simulink model "Ziegler_Nichols_PID"  (R2020b)
settings: Solver=VariableStepAuto  StartTime=0.0  StopTime=50  MaxStep=0.01  RelTol=1e-3
libraries: pid_lib x1
settings Model: Creator=amnessa  LastModifiedBy=amnessa

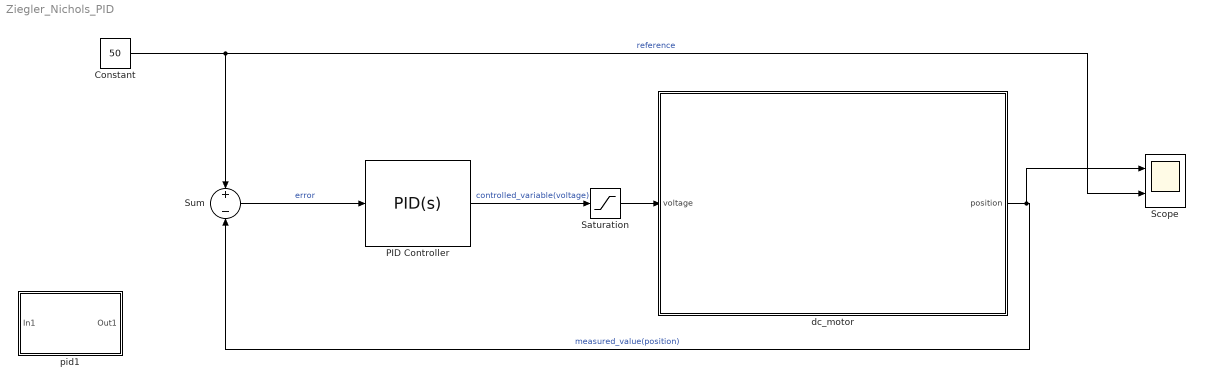
== system Ziegler_Nichols_PID ==
  Constant : Constant  Value=50
  PID Controller : pid_lib/PID Controller  Controller=PID  Form=Parallel  TimeDomain=Continuous-time  UseExternalTs=off  SampleTime=-1  IntegratorMethod=Forward Euler  FilterMethod=Forward Euler  ControllerParametersSource=internal  P=6.77668774596396  I=1.08320309237299  D=5.65172406078375  UseFilter=on  N=1208.48557960799  TunerSelectOption=Transfer Function Based (PID Tuner App)  InitialConditionSource=internal  InitialConditionForIntegrator=0  InitialConditionForFilter=0  DifferentiatorICPrevScaledInput=0  ExternalReset=none  TrackingMode=off  Kt=1  LimitOutput=off  SatLimitsSource=internal  UpperSaturationLimit=inf  LowerSaturationLimit=-inf  LinearizeAsGain=on  AntiWindupMode=none  Kb=1  POutMin=[]  POutMax=[]  IOutMin=[]  IOutMax=[]  DOutMin=[]  DOutMax=[]  NOutMin=[]  NOutMax=[]  SumOutMin=[]  SumOutMax=[]  SaturationOutMin=[]  SaturationOutMax=[]  PParamMin=[]  PParamMax=[]  IParamMin=[]  IParamMax=[]  DParamMin=[]  DParamMax=[]  NParamMin=[]  NParamMax=[]  KbParamMin=[]  KbParamMax=[]  KtParamMin=[]  KtParamMax=[]  KbOutMin=[]  KbOutMax=[]  KtOutMin=[]  KtOutMax=[]  IntegratorOutMin=[]  IntegratorOutMax=[]  FilterOutMin=[]  FilterOutMax=[]  SumI1OutMin=[]  SumI1OutMax=[]  SumI2OutMin=[]  SumI2OutMax=[]  SumI3OutMin=[]  SumI3OutMax=[]  SumI4OutMin=[]  SumI4OutMax=[]  SumDOutMin=[]  SumDOutMax=[]  DifferentiatorOutMin=[]  DifferentiatorOutMax=[]  FilterDiffOutCoefMin=[]  FilterDiffOutCoefMax=[]  ReciprocalOutMin=[]  ReciprocalOutMax=[]  SumDenOutMin=[]  SumDenOutMax=[]  SumNumOutMin=[]  SumNumOutMax=[]  DivideOutMin=[]  DivideOutMax=[]  UdiffTsProdOutMin=[]  UdiffTsProdOutMax=[]  NTsProdOutMin=[]  NTsProdOutMax=[]  UintegralTsProdOutMin=[]  UintegralTsProdOutMax=[]  UngainTsProdOutMin=[]  UngainTsProdOutMax=[]  IntegratorContinuousStateAttributes=''  IntegratorStateMustResolveToSignalObject=off  IntegratorRTWStateStorageClass=Auto  FilterContinuousStateAttributes=''  FilterStateMustResolveToSignalObject=off  FilterRTWStateStorageClass=Auto  ParallelPVariant=InternalParameters  IdealPVariant=Disabled  IVariant=InternalParameters  DVariant=InternalParameters  IntegratorVariant=Continuous  SatVariant=Disabled  AWVariant=Passthrough  PCopyVariant=Disabled  TRVariant=Disabled  FdbkBlocksVariant=Forward  IdealPFdbkVariant=Disabled  SatFdbkVariant=Disabled  DerivativeFilterVariant=ContFilter  NVariant=InternalParameters  NCopyVariant=Disabled  FilterICVariant=InternalICsFilter  IntegratorICVariant=InternalICs  ExternalResetVariant=Disabled  TRSumVariant=Passthrough  SumFdbkVariant=Disabled  SumVariant=Sum_PID  TsampFilterVariant=InternalTs  TsampNgainVariant=Passthrough  TsampIntegralVariant=Passthrough  ExternalSaturationOutDataTypeStr=Inherit: Same as second input
  Saturation : Saturate  UpperLimit=220  LowerLimit=-220
  Scope : Scope  NumInputPorts=2
  Sum : Sum  Inputs=+-
  dc_motor : Subsystem  mask{J=0.03, B=0.01, KT=0.5, R=8, L=0.45, KB=0.5}
      mask prompts: J "(J/KG*M^2)"; B "B(Nm/rad)"; KT "KT(NM/AMPER)"; R "R(OHM)"; L "L(H)"; KB "KB(Vsn/rad)"
  pid1 : Subsystem  mask{kp=175*0.6, ki=1.2*(175/1.274), kd=0.15*175*1.274}
      mask prompts: kp "proportional"; ki "integrational"; kd "derivational"
      mask DialogControl Container9 Prompt: Tab
  wires:
  dc_motor/1(position) -> Scope/1, Sum/2  "measured_value(position)"
  Constant/1 -> Scope/2, Sum/1  "reference"
  Sum/1 -> PID Controller/1  "error"
  PID Controller/1 -> Saturation/1  "controlled_variable(voltage)"
  Saturation/1 -> dc_motor/1(voltage)

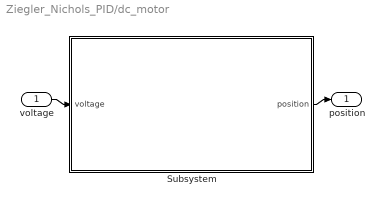
== system Ziegler_Nichols_PID/dc_motor ==
  voltage : Inport
  Subsystem : Subsystem
  position : Outport
  wires:
  Subsystem/1(position) -> position/1
  voltage/1 -> Subsystem/1(voltage)

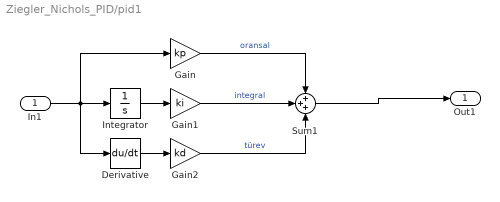
== system Ziegler_Nichols_PID/pid1 ==
  In1 : Inport
  Derivative : Derivative
  Gain : Gain  Gain=kp
  Gain1 : Gain  Gain=ki
  Gain2 : Gain  Gain=kd
  Integrator : Integrator
  Sum1 : Sum  Inputs=+++
  Out1 : Outport
  wires:
  Sum1/1 -> Out1/1
  Derivative/1 -> Gain2/1
  Gain1/1 -> Sum1/2  "integral"
  Integrator/1 -> Gain1/1
  Gain/1 -> Sum1/1  "oransal"
  Gain2/1 -> Sum1/3  "türev"
  In1/1 -> Integrator/1, Gain/1, Derivative/1

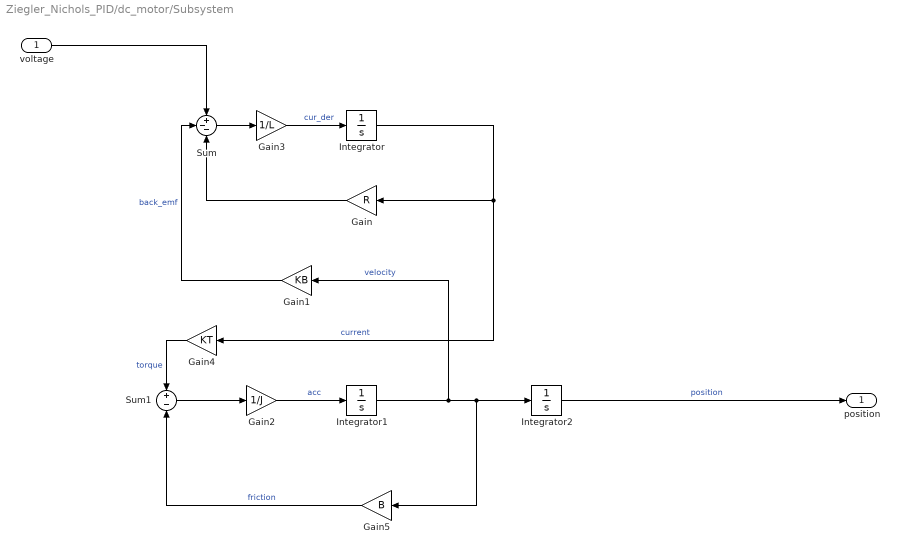
== system Ziegler_Nichols_PID/dc_motor/Subsystem ==
  voltage : Inport
  Gain : Gain  Gain=R
  Gain1 : Gain  Gain=KB
  Gain2 : Gain  Gain=1/J
  Gain3 : Gain  Gain=1/L
  Gain4 : Gain  Gain=KT
  Gain5 : Gain  Gain=B
  Integrator : Integrator
  Integrator1 : Integrator
  Integrator2 : Integrator
  Sum : Sum  Inputs=+--
  Sum1 : Sum  Inputs=+-
  position : Outport
  wires:
  Gain3/1 -> Integrator/1  "cur_der"
  Gain4/1 -> Sum1/1  "torque"
  Integrator/1 -> Gain4/1, Gain/1  "current"
  Gain2/1 -> Integrator1/1  "acc"
  Integrator1/1 -> Gain1/1, Gain5/1, Integrator2/1  "velocity"
  Sum1/1 -> Gain2/1
  Sum/1 -> Gain3/1
  Gain1/1 -> Sum/2  "back_emf"
  Gain5/1 -> Sum1/2  "friction"
  Gain/1 -> Sum/3
  Integrator2/1 -> position/1  "position"
  voltage/1 -> Sum/1
